simulink model "Xl_ch16_LPF_int_v5"  (Simulink 7.5)
settings: Solver=VariableStepDiscrete  StartTime=0.0  StopTime=0.001  RelTol=1e-3
values from neighbouring files (symbols this model uses):
  a2a = zeros(nFc, length(Hd.sosMatrix(:,5)))    [iirButter_SOS_init_v2.m]    (also in iirButter_SOS_init_v2_8pole.m)
  a3a = zeros(nFc, length(Hd.sosMatrix(:,6)))    [iirButter_SOS_init_v2.m]    (also in iirButter_SOS_init_v2_8pole.m)
  dt = 1/Fsim    (= 2.56e-06)    [iirButter_SOS_init_v2.m]    (also in iirButter_SOS_init_v2_8pole.m)
  Fc_min = 10    [iirButter_SOS_init_v2.m]    (also in iirButter_SOS_init_v2_8pole.m)
  ga = zeros(nFc, length(Hd.ScaleValues))    [iirButter_SOS_init_v2.m]    (also in iirButter_SOS_init_v2_8pole.m = zeros(nFc, length(Hd.ScaleValues(1:end-1))))
  rFc = (Fc_max/Fc_min)^(1/(nFc - 1))    (= 1.70532863139)    [iirButter_SOS_init_v2.m]    (also in iirButter_SOS_init_v2_8pole.m)
  Sra = 2^34|.02  |.027 |.027 |<.038| 1e-6|<2e-6|<2e-6|<2e-6|<2e-6| 8e-6|    [iirButter_SOS_init_v2.m]    (also in iirButter_SOS_init_v2_8pole.m)
  Srm = 2^34|     |     |     |     |     |     |     |     |     |  to |    [iirButter_SOS_init_v2.m]    (also in iirButter_SOS_init_v2_8pole.m)
libraries: xbsIndex_r4 x581, dspsrcs4 x16, simulink x8
(part 4 of 4)

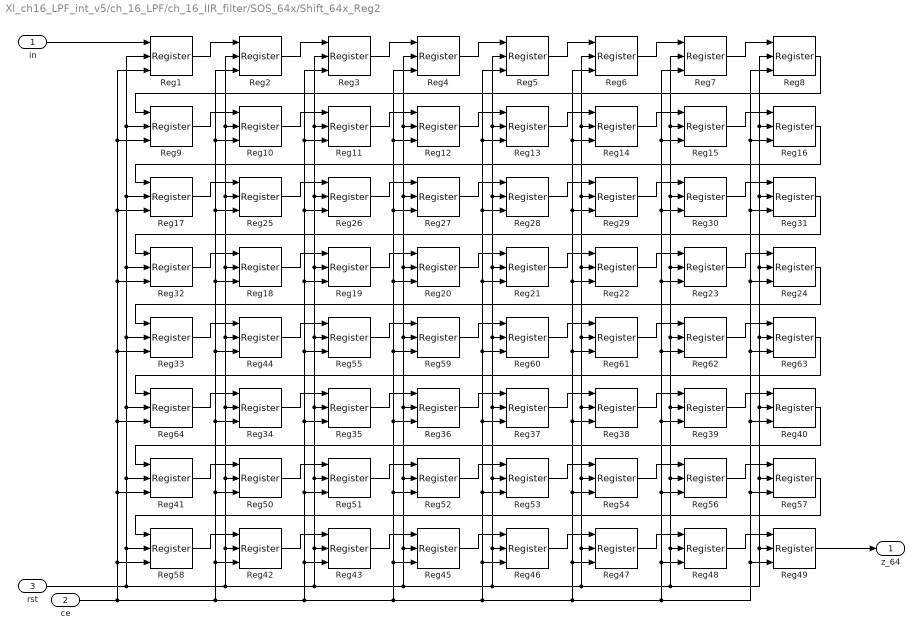
== system Xl_ch16_LPF_int_v5/ch_16_LPF/ch_16_IIR_filter/SOS_64x/Shift_64x_Reg2 ==
  in : Inport  OutDataType=fixdt(1, 16)  OutScaling=2^0
  ce : Inport  Port=2  OutDataType=fixdt(1, 16)  OutScaling=2^0
  rst : Inport  Port=3  OutDataType=fixdt(1, 16)  OutScaling=2^0
  Reg{1..64} (64 alike) : xbsIndex_r4/Register  init=0  rst=on  en=on  dbl_ovrd=off  block_type=register
      settings: block_version=12.2
  z_64 : Outport  OutDataType=fixdt(1, 16)  OutScaling=2^0
  wires:
  ce/1 -> Reg58/3, Reg41/3, Reg64/3, Reg33/3, Reg32/3, Reg17/3, Reg9/3, Reg1/3, Reg42/3, Reg50/3, Reg34/3, Reg44/3, Reg18/3, Reg25/3, Reg10/3, Reg2/3, Reg43/3, Reg51/3, Reg35/3, Reg55/3, Reg19/3, Reg26/3, Reg11/3, Reg3/3, Reg45/3, Reg52/3, Reg36/3, Reg59/3, Reg20/3, Reg27/3, Reg12/3, Reg4/3, Reg46/3, Reg53/3, Reg37/3, Reg60/3, Reg21/3, Reg28/3, Reg13/3, Reg5/3, Reg47/3, Reg54/3, Reg38/3, Reg61/3, Reg22/3, Reg29/3, Reg14/3, Reg6/3, Reg48/3, Reg56/3, Reg39/3, Reg62/3, Reg23/3, Reg30/3, Reg15/3, Reg7/3, Reg49/3, Reg57/3, Reg40/3, Reg63/3, Reg24/3, Reg31/3, Reg16/3, Reg8/3
  rst/1 -> Reg58/2, Reg41/2, Reg64/2, Reg33/2, Reg32/2, Reg17/2, Reg9/2, Reg1/2, Reg42/2, Reg50/2, Reg34/2, Reg44/2, Reg18/2, Reg25/2, Reg10/2, Reg2/2, Reg11/2, Reg3/2, Reg26/2, Reg19/2, Reg55/2, Reg35/2, Reg51/2, Reg43/2, Reg45/2, Reg52/2, Reg36/2, Reg59/2, Reg20/2, Reg27/2, Reg12/2, Reg4/2, Reg46/2, Reg53/2, Reg37/2, Reg60/2, Reg21/2, Reg28/2, Reg13/2, Reg5/2, Reg47/2, Reg54/2, Reg38/2, Reg61/2, Reg22/2, Reg29/2, Reg14/2, Reg6/2, Reg48/2, Reg56/2, Reg39/2, Reg62/2, Reg23/2, Reg30/2, Reg15/2, Reg7/2, Reg49/2, Reg57/2, Reg40/2, Reg63/2, Reg24/2, Reg31/2, Reg16/2, Reg8/2
  Reg49/1 -> z_64/1
  Reg24/1 -> Reg33/1
  Reg40/1 -> Reg41/1
  Reg57/1 -> Reg58/1
  Reg58/1 -> Reg42/1
  Reg42/1 -> Reg43/1
  Reg43/1 -> Reg45/1
  Reg45/1 -> Reg46/1
  Reg46/1 -> Reg47/1
  Reg47/1 -> Reg48/1
  Reg48/1 -> Reg49/1
  Reg41/1 -> Reg50/1
  Reg50/1 -> Reg51/1
  Reg51/1 -> Reg52/1
  Reg52/1 -> Reg53/1
  Reg53/1 -> Reg54/1
  Reg54/1 -> Reg56/1
  Reg56/1 -> Reg57/1
  Reg63/1 -> Reg64/1
  Reg64/1 -> Reg34/1
  Reg34/1 -> Reg35/1
  Reg35/1 -> Reg36/1
  Reg36/1 -> Reg37/1
  Reg37/1 -> Reg38/1
  Reg38/1 -> Reg39/1
  Reg39/1 -> Reg40/1
  Reg33/1 -> Reg44/1
  Reg44/1 -> Reg55/1
  Reg55/1 -> Reg59/1
  Reg59/1 -> Reg60/1
  Reg60/1 -> Reg61/1
  Reg61/1 -> Reg62/1
  Reg62/1 -> Reg63/1
  Reg16/1 -> Reg17/1
  Reg31/1 -> Reg32/1
  Reg32/1 -> Reg18/1
  Reg18/1 -> Reg19/1
  Reg19/1 -> Reg20/1
  Reg20/1 -> Reg21/1
  Reg21/1 -> Reg22/1
  Reg22/1 -> Reg23/1
  Reg23/1 -> Reg24/1
  Reg17/1 -> Reg25/1
  Reg25/1 -> Reg26/1
  Reg26/1 -> Reg27/1
  Reg27/1 -> Reg28/1
  Reg28/1 -> Reg29/1
  Reg29/1 -> Reg30/1
  Reg30/1 -> Reg31/1
  Reg8/1 -> Reg9/1
  Reg9/1 -> Reg10/1
  Reg10/1 -> Reg11/1
  Reg11/1 -> Reg12/1
  Reg12/1 -> Reg13/1
  Reg13/1 -> Reg14/1
  Reg14/1 -> Reg15/1
  Reg15/1 -> Reg16/1
  in/1 -> Reg1/1
  Reg1/1 -> Reg2/1
  Reg2/1 -> Reg3/1
  Reg3/1 -> Reg4/1
  Reg4/1 -> Reg5/1
  Reg5/1 -> Reg6/1
  Reg6/1 -> Reg7/1
  Reg7/1 -> Reg8/1

== system Xl_ch16_LPF_int_v5/ch_16_LPF/ch_16_IIR_filter/SOS_64x_IO_ctrl/ch_16_filt_sync ==
  note: Keep fsync phase consistent
      | with gc/a2c/a3c  phase
  cnt6b : Inport  OutDataType=fixdt(1, 16)  OutScaling=2^0
  AeqB : xbsIndex_r4/Relational  mode=a=b  en=off  latency=0  dbl_ovrd=off  block_type=relational
      settings: block_version=12.2
  Constant : xbsIndex_r4/Constant  arith_type=Unsigned  const=2  n_bits=2  bin_pt=0  explicit_period=off  period=1  equ=P=C  opselect=C  inp2=PCIN>>17  opr=+  inp1=P  carry=CIN  dbl_ovrd=off  block_type=constant
      settings: block_version=12.2
  Slice_2LSB : xbsIndex_r4/Slice  nbits=2  boolean_output=off  mode=Lower Bit Location + Width  bit1=0  base1=MSB of Input  bit0=0  base0=LSB of Input  dbl_ovrd=off  block_type=slice
      settings: block_version=12.2
  fsync : Outport  OutDataType=fixdt(1, 16)  OutScaling=2^0
  wires:
  cnt6b/1 -> Slice_2LSB/1
  Slice_2LSB/1 -> AeqB/1
  AeqB/1 -> fsync/1
  Constant/1 -> AeqB/2

== system Xl_ch16_LPF_int_v5/ch_16_LPF/ch_16_IIR_filter/SOS_64x_IO_ctrl/ch_16_filt_sync1 ==
  note: Keep fsync phase consistent
      | with gc/a2c/a3c  phase
  cnt6b : Inport  OutDataType=fixdt(1, 16)  OutScaling=2^0
  AeqB : xbsIndex_r4/Relational  mode=a=b  en=off  latency=0  dbl_ovrd=off  block_type=relational
      settings: block_version=12.2
  Constant : xbsIndex_r4/Constant  arith_type=Unsigned  const=3  n_bits=2  bin_pt=0  explicit_period=off  period=1  equ=P=C  opselect=C  inp2=PCIN>>17  opr=+  inp1=P  carry=CIN  dbl_ovrd=off  block_type=constant
      settings: block_version=12.2
  Slice_2LSB : xbsIndex_r4/Slice  nbits=2  boolean_output=off  mode=Lower Bit Location + Width  bit1=0  base1=MSB of Input  bit0=0  base0=LSB of Input  dbl_ovrd=off  block_type=slice
      settings: block_version=12.2
  fsync : Outport  OutDataType=fixdt(1, 16)  OutScaling=2^0
  wires:
  cnt6b/1 -> Slice_2LSB/1
  Slice_2LSB/1 -> AeqB/1
  AeqB/1 -> fsync/1
  Constant/1 -> AeqB/2

== system Xl_ch16_LPF_int_v5/ch_16_LPF/ch_16_IIR_filter/Demux_16x/dec_4bit/bus2bit ==
  d : Inport
  extraxt_b0 : xbsIndex_r4/Slice  nbits=1  boolean_output=on  mode=Lower Bit Location + Width  bit1=0  base1=MSB of Input  bit0=0  base0=LSB of Input  dbl_ovrd=off  block_type=slice
      settings: block_version=12.2
  extraxt_b1 : xbsIndex_r4/Slice  nbits=1  boolean_output=on  mode=Lower Bit Location + Width  bit1=0  base1=MSB of Input  bit0=1  base0=LSB of Input  dbl_ovrd=off  block_type=slice
      settings: block_version=12.2
  extraxt_b2 : xbsIndex_r4/Slice  nbits=1  boolean_output=on  mode=Lower Bit Location + Width  bit1=0  base1=MSB of Input  bit0=2  base0=LSB of Input  dbl_ovrd=off  block_type=slice
      settings: block_version=12.2
  extraxt_b3 : xbsIndex_r4/Slice  nbits=1  boolean_output=on  mode=Lower Bit Location + Width  bit1=0  base1=MSB of Input  bit0=3  base0=LSB of Input  dbl_ovrd=off  block_type=slice
      settings: block_version=12.2
  b0 : Outport
  b1 : Outport  Port=2
  b2 : Outport  Port=3
  b3 : Outport  Port=4
  wires:
  d/1 -> extraxt_b0/1, extraxt_b1/1, extraxt_b3/1, extraxt_b2/1
  extraxt_b0/1 -> b0/1
  extraxt_b1/1 -> b1/1
  extraxt_b2/1 -> b2/1
  extraxt_b3/1 -> b3/1

== system Xl_ch16_LPF_int_v5/ch_16_LPF/ch_16_IIR_filter/Demux_16x/dec_4bit/neg_bus2bit ==
  d : Inport
  extraxt_b0 : xbsIndex_r4/Slice  nbits=1  boolean_output=on  mode=Lower Bit Location + Width  bit1=0  base1=MSB of Input  bit0=0  base0=LSB of Input  dbl_ovrd=off  block_type=slice
      settings: block_version=12.2
  extraxt_b1 : xbsIndex_r4/Slice  nbits=1  boolean_output=on  mode=Lower Bit Location + Width  bit1=0  base1=MSB of Input  bit0=1  base0=LSB of Input  dbl_ovrd=off  block_type=slice
      settings: block_version=12.2
  extraxt_b2 : xbsIndex_r4/Slice  nbits=1  boolean_output=on  mode=Lower Bit Location + Width  bit1=0  base1=MSB of Input  bit0=2  base0=LSB of Input  dbl_ovrd=off  block_type=slice
      settings: block_version=12.2
  extraxt_b3 : xbsIndex_r4/Slice  nbits=1  boolean_output=on  mode=Lower Bit Location + Width  bit1=0  base1=MSB of Input  bit0=3  base0=LSB of Input  dbl_ovrd=off  block_type=slice
      settings: block_version=12.2
  b0 : Outport
  b1 : Outport  Port=2
  b2 : Outport  Port=3
  b3 : Outport  Port=4
  wires:
  extraxt_b3/1 -> b3/1
  extraxt_b2/1 -> b2/1
  extraxt_b1/1 -> b1/1
  extraxt_b0/1 -> b0/1
  d/1 -> extraxt_b2/1, extraxt_b3/1, extraxt_b1/1, extraxt_b0/1
